simulink model "pitch"  (R2023a)
settings: Solver=VariableStepAuto  StartTime=0.0  StopTime=10  RelTol=1e-3
values from neighbouring files (symbols this model uses):
  A_long = inv(P_long) * Q_long    [parameters_ctrl.m]
  B_long = inv(P_long) * R_long    [parameters_ctrl.m]
  C_long = eye(4)    [parameters_ctrl.m]
  CNh0 = 0.2835    [parameters_ctrl.m]
  CNw = 0.82    [parameters_ctrl.m]
  D_long = zeros(4,2)    [parameters_ctrl.m]
  dclddc = 0.22    [parameters_ctrl.m]
  rho = 1.225    [parameters_ctrl.m]
  S = 0.76    [parameters_ctrl.m]
  Sh = 0.123708    [parameters_ctrl.m]
  V = 15.1    [parameters_ctrl.m]
  W = mass * g    (= 86.9166)    [parameters_ctrl.m]
settings Model: Creator=simon  LastModifiedBy=simon

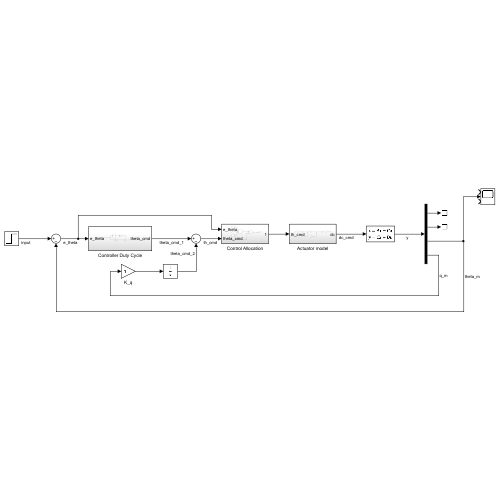
[thumbnail: Simulink's stored preview of the top-level diagram]
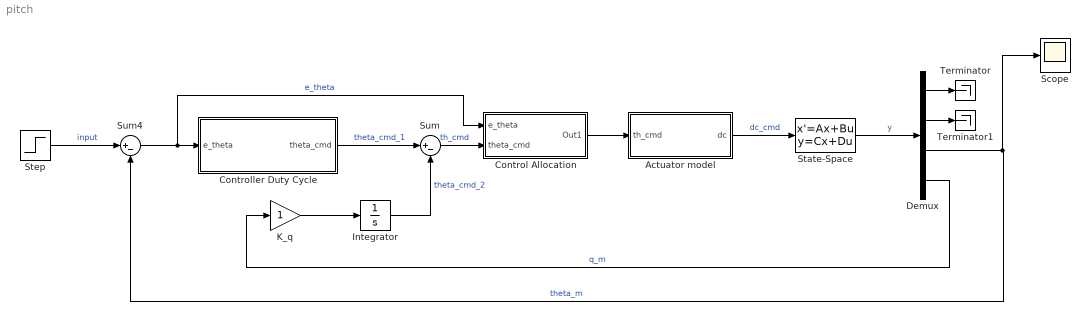
== system pitch ==
  Actuator model : Subsystem
  Control Allocation : Subsystem
  Controller Duty Cycle : Subsystem
  Demux : Demux
  Integrator : Integrator
  K_q : Gain
  Scope : Scope  NumInputPorts=3
  State-Space : StateSpace  A=A_long  B=B_long  C=C_long  D=D_long  InitialCondition=0
  Step : Step  After=0.02  SampleTime=0
  Sum : Sum  Inputs=|+-
  Sum4 : Sum  Inputs=|+-
  Terminator : Terminator
  Terminator1 : Terminator
  wires:
  Step/1 -> Sum4/1  "input"
  Sum4/1 -> Control Allocation/1(e_theta), Controller Duty Cycle/1(e_theta)  "e_theta"
  Demux/3 -> Scope/2, Sum4/2  "theta_m"
  Actuator model/1(dc) -> State-Space/1  "dc_cmd"
  Controller Duty Cycle/1(theta_cmd) -> Sum/1  "theta_cmd_1"
  Control Allocation/1(Out1) -> Actuator model/1(th_cmd)
  State-Space/1 -> Demux/1  "y"
  Demux/1 -> Terminator/1
  Demux/2 -> Terminator1/1
  K_q/1 -> Integrator/1
  Integrator/1 -> Sum/2  "theta_cmd_2"
  Demux/4 -> K_q/1  "q_m"
  Sum/1 -> Control Allocation/2(theta_cmd)  "th_cmd"

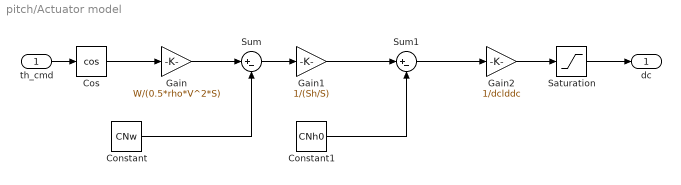
== system pitch/Actuator model ==
  th_cmd : Inport
  Constant : Constant  Value=CNw
  Constant1 : Constant  Value=CNh0
  Cos : Trigonometry  Operator=cos
  Gain : Gain  Gain=W/(0.5*rho*V^2*S)
  Gain1 : Gain  Gain=1/(Sh/S)
  Gain2 : Gain  Gain=1/dclddc
  Saturation : Saturate  UpperLimit=1  LowerLimit=0
  Sum : Sum  Inputs=|+-
  Sum1 : Sum  Inputs=|+-
  dc : Outport
  wires:
  th_cmd/1 -> Cos/1
  Cos/1 -> Gain/1
  Constant/1 -> Sum/2
  Gain/1 -> Sum/1
  Sum/1 -> Gain1/1
  Gain1/1 -> Sum1/1
  Constant1/1 -> Sum1/2
  Sum1/1 -> Gain2/1
  Gain2/1 -> Saturation/1
  Saturation/1 -> dc/1

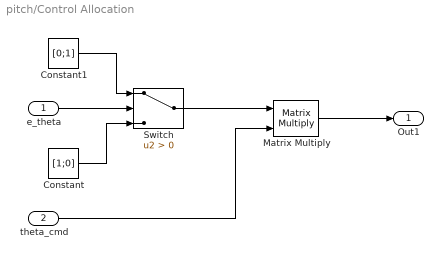
== system pitch/Control Allocation ==
  e_theta : Inport
  theta_cmd : Inport  Port=2
  Constant : Constant  Value=[1;0]  VectorParams1D=off
  Constant1 : Constant  Value=[0;1]  VectorParams1D=off
  Matrix Multiply : Product  Multiplication=Matrix(*)
  Switch : Switch  Criteria=u2 > Threshold  SaturateOnIntegerOverflow=off  InputSameDT=off
  Out1 : Outport
  wires:
  Matrix Multiply/1 -> Out1/1
  theta_cmd/1 -> Matrix Multiply/2
  e_theta/1 -> Switch/2
  Constant/1 -> Switch/3
  Constant1/1 -> Switch/1
  Switch/1 -> Matrix Multiply/1

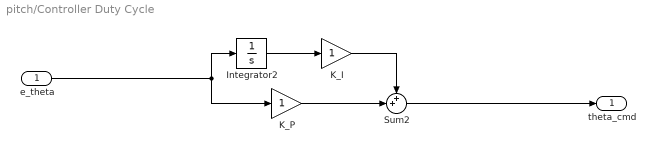
== system pitch/Controller Duty Cycle ==
  e_theta : Inport
  Integrator2 : Integrator
  K_I : Gain
  K_P : Gain
  Sum2 : Sum  Inputs=++|
  theta_cmd : Outport
  wires:
  e_theta/1 -> K_P/1, Integrator2/1
  K_I/1 -> Sum2/1
  K_P/1 -> Sum2/2
  Integrator2/1 -> K_I/1
  Sum2/1 -> theta_cmd/1
